simulink model "controllo_ss_PP_Luenberger"  (R2023b)
settings: Solver=VariableStepAuto  StartTime=0.0  StopTime=20  RelTol=1e-3
values from neighbouring files (symbols this model uses):
  A_ob = A - L_kf*C    [LQ_KF_version1.m]    (also in LQ_KF_version2.m; LQ_Luenberger.m; PP_Luenberger.m = A - L*C; prova1.m = A - L*C)
  B_ob = [ B - L_kf*D, L_kf]    [LQ_KF_version1.m]    (also in LQ_KF_version2.m; LQ_Luenberger.m; PP_Luenberger.m = [ B, L]; prova1.m = [ B, L])
  C_ob = eye(n)    [LQ_KF_version1.m]    (also in LQ_KF_version2.m; LQ_Luenberger.m; PP_Luenberger.m; prova1.m)
  D_ob = zeros(n, m+p)    [LQ_KF_version1.m]    (also in LQ_KF_version2.m; LQ_Luenberger.m; PP_Luenberger.m; prova1.m)
  Ken_eta = K(:, 4)    [LQ_KF_version1.m]    (also in LQ_KF_version2.m = Ken(:, n+1:end); LQ_Luenberger.m; PP_Luenberger.m = Ken(:, n+1:end); prova1.m = Ken(:, n+1:end))
  Ken_x = K(:, 1:3)    [LQ_KF_version1.m]    (also in LQ_KF_version2.m = Ken(:, 1:n); LQ_Luenberger.m; PP_Luenberger.m = Ken(:, 1:n); prova1.m = Ken(:, 1:n))
undefined symbols (not defined in the file or in its folder): Lc, Rtot, x1_eq0, x2_eq0
libraries: simulink x1
settings Model: Creator=Pronto all'uso  LastModifiedBy=Pronto all'uso

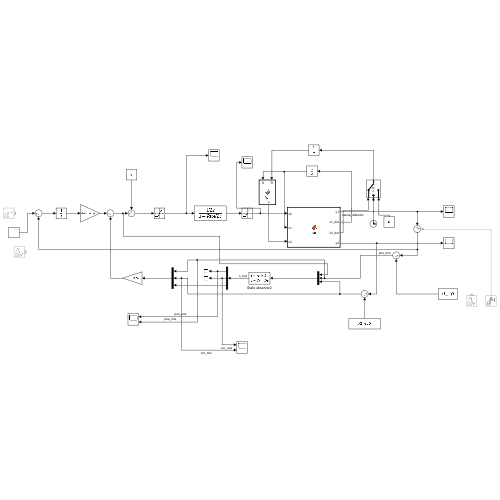
[thumbnail: Simulink's stored preview of the top-level diagram]
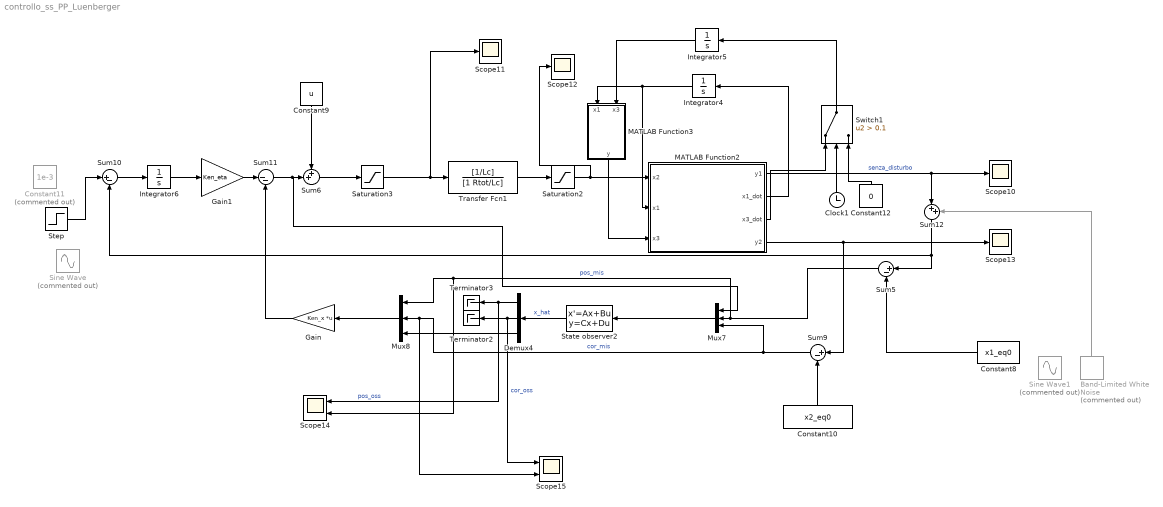
== system controllo_ss_PP_Luenberger ==
  Band-Limited White Noise : simulink/Sources/Band-Limited White Noise  Commented=on  Cov=[8.9934e-11*0.002]  Ts=0.002  seed=[23341]
  Clock1 : Clock
  Constant10 : Constant  Value=x2_eq0
  Constant11 : Constant  Commented=on  Value=1e-3
  Constant12 : Constant  Value=0
  Constant8 : Constant  Value=x1_eq0
  Constant9 : Constant  Value=u
  Demux4 : Demux  Outputs=3
  Gain : Gain  Gain=Ken_x  Multiplication=Matrix(K*u)
  Gain1 : Gain  Gain=Ken_eta
  Integrator4 : Integrator  InitialCondition=x1_eq0
  Integrator5 : Integrator
  Integrator6 : Integrator
  MATLAB Function2 : MATLAB Function  TreatAsAtomicUnit=on
  MATLAB Function3 : MATLAB Function  TreatAsAtomicUnit=on
  Mux7 : Mux  Inputs=3
  Mux8 : Mux  Inputs=3
  Saturation2 : Saturate  UpperLimit=3  LowerLimit=0
  Saturation3 : Saturate  UpperLimit=24  LowerLimit=-24
  Scope{10..13} (4 alike) : Scope
  Scope14 : Scope  NumInputPorts=2
  Scope15 : Scope  NumInputPorts=2
  Sine Wave : Sin  Commented=on  Amplitude=0.002  Bias=0.004  Frequency=10  SampleTime=0
  Sine Wave1 : Sin  Commented=on  Amplitude=0.0001  Frequency=200  SampleTime=0.002
  State observer2 : StateSpace  A=A_ob  B=B_ob  C=C_ob  D=D_ob  InitialCondition=[0;0;0]  ParameterTunability=Unconstrained
  Step : Step  Time=3  Before=-0.001  After=0.001  SampleTime=0
  Sum10 : Sum  Inputs=|+-
  Sum11 : Sum  Inputs=|--
  Sum12 : Sum  Inputs=|++
  Sum5 : Sum  Inputs=|+-
  Sum6 : Sum  Inputs=++|
  Sum9 : Sum  Inputs=|+-
  Switch1 : Switch  Criteria=u2 > Threshold  Threshold=0.1  SaturateOnIntegerOverflow=off  InputSameDT=off
  Terminator2 : Terminator
  Terminator3 : Terminator
  Transfer Fcn1 : TransferFcn  Numerator=[1/Lc]  Denominator=[1 Rtot/Lc]
  wires:
  MATLAB Function2/2(x1_dot) -> Integrator4/1
  Integrator4/1 -> MATLAB Function2/2(x1), MATLAB Function3/1(x1)
  Integrator5/1 -> MATLAB Function3/2(x3)
  Transfer Fcn1/1 -> Saturation2/1
  Saturation2/1 -> MATLAB Function2/1(x2), Scope12/1
  MATLAB Function2/1(y1) -> Sum12/1, Scope10/1  "senza_disturbo"
  Constant8/1 -> Sum5/2
  Sum6/1 -> Saturation3/1
  Constant9/1 -> Sum6/1
  Mux7/1 -> State observer2/1
  Sum5/1 -> Scope14/2, Mux8/1, Mux7/2  "pos_mis"
  Constant10/1 -> Sum9/2
  Sum9/1 -> Scope15/2, Mux8/2, Mux7/3  "cor_mis"
  Gain1/1 -> Sum11/1
  Gain/1 -> Sum11/2
  Integrator6/1 -> Gain1/1
  Sum10/1 -> Integrator6/1
  MATLAB Function3/1(y) -> MATLAB Function2/3(x3)
  MATLAB Function2/4(y2) -> Sum9/1, Scope13/1
  Sum11/1 -> Mux7/1, Sum6/2
  MATLAB Function2/3(x3_dot) -> Switch1/1
  Switch1/1 -> Integrator5/1
  Constant12/1 -> Switch1/3
  Clock1/1 -> Switch1/2
  Saturation3/1 -> Transfer Fcn1/1, Scope11/1
  State observer2/1 -> Demux4/1  "x_hat"
  Mux8/1 -> Gain/1
  Demux4/3 -> Mux8/3
  Demux4/1 -> Scope14/1, Terminator3/1  "pos_oss"
  Demux4/2 -> Scope15/1, Terminator2/1  "cor_oss"
  Sum12/1 -> Sum10/2, Sum5/1
  Step/1 -> Sum10/1
  Band-Limited White Noise/1 -> Sum12/2

== matlab function controllo_ss_PP_Luenberger/MATLAB Function2 ==
  data: y1 output; x2 input; x1_dot output; x1 input; x3 input; x3_dot output; y2 output
function [y1,x1_dot, x3_dot, y2] = fcn(x2, x1, x3)
    m = 0.0657;
    g = 9.81;
    k_mag = 2.4405e-05;
    Rtot = 9.7585;
    Lc = 0.3708;
    y0 = 0.012;
    
    x1_dot = x3;
    x3_dot = (k_mag/m)*(x2/(y0-x1))^2 - g;
y1 = x1;
y2 = x2;

== matlab function controllo_ss_PP_Luenberger/MATLAB Function3 ==
  data: x1 input; y output; x3 input
function y = fcn(x1,x3)
if x1 <= 0
    x3 = 0;
end
y = x3;
